simulink model "BDC_prototype"  (R2019a)
settings: Solver=VariableStepAuto  StartTime=0.0  StopTime=10.0  RelTol=1e-3
values from neighbouring files (symbols this model uses):
  sample_time = Ts    (= 0.0001)    [current_digital_control.m]    (also in voltage_digital_control.m)
undefined symbols (not defined in the file or in its folder): Ion, Lithium
libraries: powerlib x52, electricdrivelib x2, simulink x2, simulink_extras x1
settings Model: Creator=kagom  LastModifiedBy=kagom
settings SolverCC: ZeroCrossAlgorithm=Adaptive  AlgebraicLoopSolver=LineSearch
settings DebuggingCC: IgnoredZcDiagnostic=none

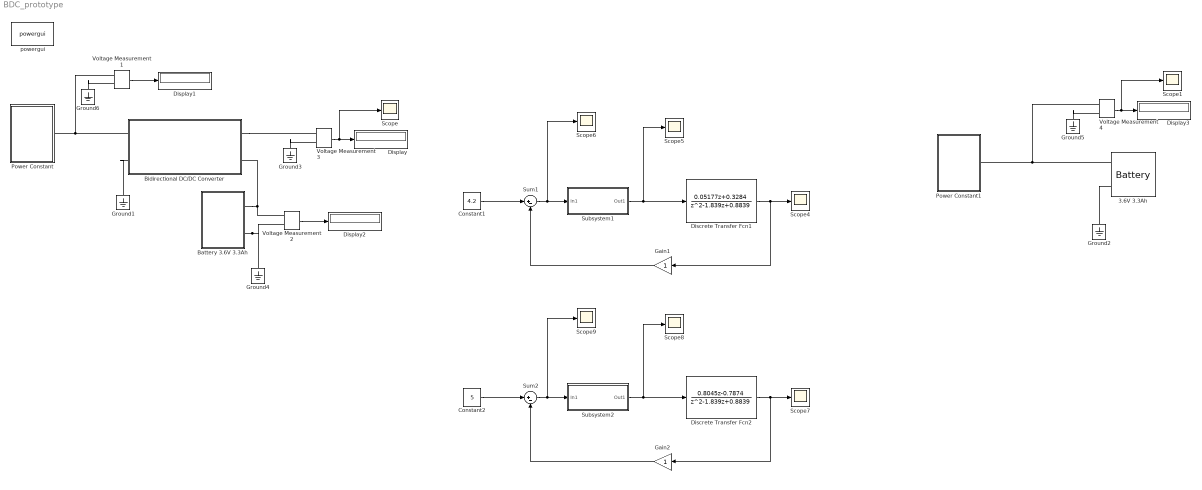
== system BDC_prototype ==
  3.6V 3.3Ah : electricdrivelib/Extra Sources/Battery  BatType=Lithium-Ion  ShowTempParam=off  ThermalPreset=no  ShowAgeParam=off  NomV=3.6  NomQ=3.3  SOC=20  Batt_Tr=1  PresetModel=on  MaxQ=3.3  MinV=2.7  FullV=4.1904  Dis_rate=1.4348  R=0.010909  Normal_OP=2.9843  expZone="[3.8894     0.16213]"  current=[6.5 13 32.5]  Units=Ampere-hour  Tci=20  NomT=20  T2=-30  MaxQ2=4.8  FullV2=7.1  Normal_OP2=5.655  expZone2="[6.58           1]"  Rca=0.6  ti=2000  Dp=0  Neq0=0  Tsim=1e6  Ta1=25  Qeol=5.4*0.9  Reol=0.013333*1.2  Char_age=[2.3478, 3]  Dis_age=[2.3478, 10]  N1=1500  N2=10500  N3=1000  N4=1400  Ta2=45  N5=950
      settings: SourceProductName=Simscape Electrical
  Battery 3.6V 3.3Ah : Subsystem
  Bidirectional DC/DC Converter : Subsystem
  Constant1 : Constant  Value=4.2  VectorParams1D=off
  Constant2 : Constant  Value=5  VectorParams1D=off
  Discrete Transfer Fcn1 : DiscreteTransferFcn  Numerator=[0.05177 0.3284]  Denominator=[1 -1.839 0.8839]
  Discrete Transfer Fcn2 : DiscreteTransferFcn  Numerator=[0.8045 -0.7874]  Denominator=[1 -1.839 0.8839]
  Display{,1..3} (4 alike) : Display
  Gain1 : Gain
  Gain2 : Gain
  Ground{1..6} (6 alike) : powerlib/Elements/Ground  LConnTagsString=a
      settings: SourceProductName=Simscape Electrical
  Power Constant : Subsystem
  Power Constant1 : Subsystem
  Scope{,1,4..9} (8 alike) : Scope
  Subsystem1 : Subsystem
  Subsystem2 : Subsystem
  Sum1 : Sum  Inputs=|+-
  Sum2 : Sum  Inputs=|+-
  Voltage Measurement{1..4} (4 alike) : powerlib/Measurements/Voltage Measurement  PhasorSimulation=off  OutputType=Complex  PSBequivalent=0
      settings: SourceProductName=Simscape Electrical
  powergui : powerlib/powergui  Priority=1  SimulationMode=Discrete  SampleTime=8e-6  frequency=60  Iterations=50  frequencyindice=0  Pbase=100e6  ErrMax=1e-4  UnitsV=kV  UnitsW=MW  buscounter=0  FunctionMessages=off  echomessages=off  EnableUseOfTLC=off  CurrentSourceSwitches=off  DisableSnubberDevices=off  DisableRonSwitches=off  DisableVfSwitches=off  DisplayEquations=off  AutomaticDiscreteSolvers=off  SolverType=Tustin/Backward Euler (TBE)  Interpol=off  ExternalGateDelay=off  methode=off  Ts=100  x0status=blocks  SPID=on  SwTol=0  HookPort=off  NonlinearTolerance=0  nMaxIteration=15  ContinueOnMaxIteration=off  RestoreLinks=warning  ResistiveCurrentMeasurement=off  Frange=[0:2:500]  Ylog=off  Xlog=on  ShowGrid=off  save=off  variable=ZData  structure=0  ZoomFFT=off  StartTime=0.0  cycles=1  DisplayStyle=1  fundamental=60  FreqAxis=off  MaxFrequency=1000  frequencyindicesteady=1  RmsSteady=1  display=off
      settings: SourceProductName=Simscape Electrical
  wires:
  Voltage Measurement1/1 -> Display1/1
  Voltage Measurement2/1 -> Display2/1
  Voltage Measurement3/1 -> Scope/1, Display/1
  Discrete Transfer Fcn1/1 -> Scope4/1, Gain1/1
  Gain1/1 -> Sum1/2
  Subsystem1/1(Out1) -> Scope5/1, Discrete Transfer Fcn1/1
  Sum1/1 -> Scope6/1, Subsystem1/1(In1)
  Constant1/1 -> Sum1/1
  Discrete Transfer Fcn2/1 -> Scope7/1, Gain2/1
  Subsystem2/1(Out1) -> Scope8/1, Discrete Transfer Fcn2/1
  Sum2/1 -> Scope9/1, Subsystem2/1(In1)
  Gain2/1 -> Sum2/2
  Constant2/1 -> Sum2/1
  Voltage Measurement4/1 -> Scope1/1, Display3/1
  connections:
  Voltage Measurement2/LConn1 -- Battery 3.6V 3.3Ah/RConn1 -- Bidirectional DC/DC Converter/RConn2
  Voltage Measurement1/LConn1 -- Bidirectional DC/DC Converter/LConn1 -- Power Constant/RConn1
  Battery 3.6V 3.3Ah/RConn2 -- Ground4/LConn1 -- Voltage Measurement2/LConn2
  Bidirectional DC/DC Converter/RConn1 -- Voltage Measurement3/LConn1
  Bidirectional DC/DC Converter/LConn2 -- Ground1/LConn1
  Ground6/LConn1 -- Voltage Measurement1/LConn2
  Ground3/LConn1 -- Voltage Measurement3/LConn2
  3.6V 3.3Ah/LConn1 -- Voltage Measurement4/LConn1 -- Power Constant1/RConn1
  Ground2/LConn1 -- 3.6V 3.3Ah/LConn2
  Ground5/LConn1 -- Voltage Measurement4/LConn2

== system BDC_prototype/Battery 3.6V 3.3Ah ==
  3.6V 3.3Ah : electricdrivelib/Extra Sources/Battery  BatType=Lithium-Ion  ShowTempParam=off  ThermalPreset=no  ShowAgeParam=off  NomV=3.6  NomQ=3.3  SOC=20  Batt_Tr=1  PresetModel=on  MaxQ=3.3  MinV=2.7  FullV=4.1904  Dis_rate=1.4348  R=0.010909  Normal_OP=2.9843  expZone="[3.8894     0.16213]"  current=[6.5 13 32.5]  Units=Ampere-hour  Tci=20  NomT=20  T2=-30  MaxQ2=4.8  FullV2=7.1  Normal_OP2=5.655  expZone2="[6.58           1]"  Rca=0.6  ti=2000  Dp=0  Neq0=0  Tsim=1e6  Ta1=25  Qeol=5.4*0.9  Reol=0.013333*1.2  Char_age=[2.3478, 3]  Dis_age=[2.3478, 10]  N1=1500  N2=10500  N3=1000  N4=1400  Ta2=45  N5=950
      settings: SourceProductName=Simscape Electrical
  Demux : Demux  Outputs=3
  + : PMIOPort  Side=Right
  GND : PMIOPort  Port=2  Side=Right
  tag scope: A=global, SOC=global, V=global
  wires:
  Demux/3 -> [V]
  3.6V 3.3Ah/1 -> Demux/1
  Demux/1 -> [SOC]
  Demux/2 -> [A]
  connections:
  3.6V 3.3Ah/LConn1 -- +/RConn1
  3.6V 3.3Ah/LConn2 -- GND/RConn1

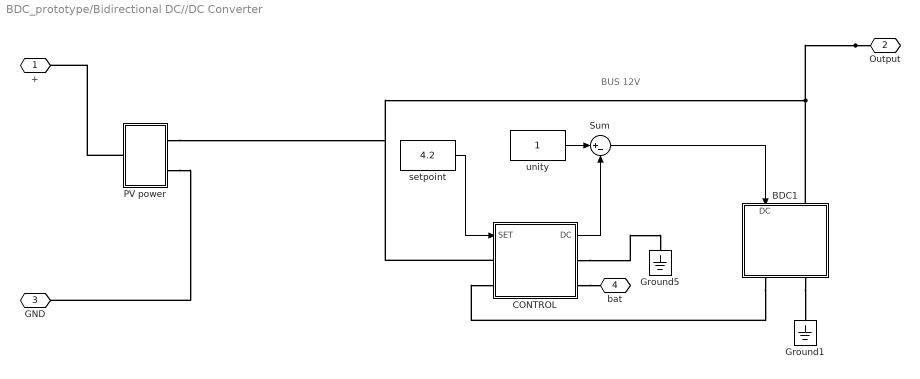
== system BDC_prototype/Bidirectional DC//DC Converter ==
  note: BUS 12V
  BDC1 : Subsystem  mask(BDC model){Ron=0.04, VD=1.5, RD=0.05, freq=125e3, tdead=19.125e-9, InputVariableName=bdc_in, OutputVariableName=bdc_out, SampleTime=sample_time}
      mask prompts: Ron "Mosfet On Resistance (Ohms)"; VD "Diode forward voltage (V)"; RD "Diode on resistance (Ohms)"; freq "Converter switching frequency (Hz)"; tdead "Driver dead time (s)"; InputVariableName "Input measurements variable name"; OutputVariableName "Output measurements variable name"; SampleTime "Simulink:blkprm_prompts:AllBlksSampleTime"
      mask help: Half-bridge averaged model with averaged losses.
      mask TypeOptions Ron: Driving Mosfet Loss/Ron | Sincronous Mosfet Loss/Ron
      mask TypeOptions VD: Diode Foward Voltage/VD
      mask TypeOptions RD: Diode On Resistance/RD
      mask TypeOptions freq:
      | Timing/fs/Value | Reverse Recovery
      | Loss of Lower Diode/freq | Reverse Recovery
      | Loss of Upper Diode/freq
      mask TypeOptions tdead: Timing/tdead/Value
      mask TypeOptions InputVariableName: Input_power/To Workspace/VariableName
      mask TypeOptions OutputVariableName: Output_power/To Workspace/VariableName
      mask TypeOptions SampleTime: Input_power/To Workspace/SampleTime | Output_power/To Workspace/SampleTime
      mask DialogControl Container9 Prompt: Logging
      mask DialogControl SampleTime Prompt: Sample time (-1 for inherited):
  CONTROL : Subsystem
  Ground1 : powerlib/Elements/Ground  LConnTagsString=a
      settings: SourceProductName=Simscape Electrical
  Ground5 : powerlib/Elements/Ground  LConnTagsString=a
      settings: SourceProductName=Simscape Electrical
  PV power : Subsystem
  Sum : Sum  Inputs=|+-
  setpoint : Constant  Value=4.2
  unity : Constant
  + : PMIOPort  Side=Left
  Output : PMIOPort  Port=2  Side=Right
  GND : PMIOPort  Port=3  Side=Left
  bat : PMIOPort  Port=4  Side=Right
  wires:
  setpoint/1 -> CONTROL/1(SET)
  Sum/1 -> BDC1/1(DC)
  CONTROL/1(DC) -> Sum/2
  unity/1 -> Sum/1
  connections:
  Output/RConn1 -- BDC1/LConn1 -- PV power/RConn1 -- CONTROL/LConn1
  CONTROL/RConn1 -- Ground5/LConn1
  BDC1/RConn2 -- Ground1/LConn1
  PV power/LConn1 -- +/RConn1
  PV power/RConn2 -- GND/RConn1
  BDC1/RConn1 -- CONTROL/LConn2
  CONTROL/RConn2 -- bat/RConn1

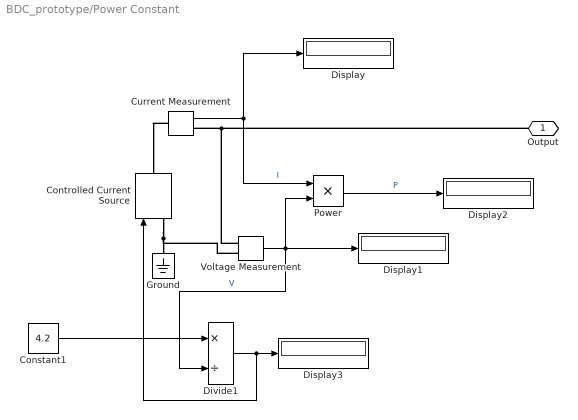
== system BDC_prototype/Power Constant ==
  Constant1 : Constant  Value=4.2  VectorParams1D=off
  Controlled Current Source : powerlib/Electrical Sources/Controlled Current Source  Initialize=on  Source_Type=DC  Amplitude=1  Phase=0  Frequency=0  Measurements=Current
      settings: SourceProductName=Simscape Electrical
  Current Measurement : powerlib/Measurements/Current Measurement  PhasorSimulation=off  OutputType=Complex  PSBequivalent=0
      settings: SourceProductName=Simscape Electrical
  Display{,1..3} (4 alike) : Display
  Divide1 : Product  Inputs=*/
  Ground : powerlib/Elements/Ground  LConnTagsString=a
      settings: SourceProductName=Simscape Electrical
  Power : Product
  Voltage Measurement : powerlib/Measurements/Voltage Measurement  PhasorSimulation=off  OutputType=Complex  PSBequivalent=0
      settings: SourceProductName=Simscape Electrical
  Output : PMIOPort  Side=Right
  wires:
  Voltage Measurement/1 -> Power/2, Divide1/2, Display1/1  "V"
  Current Measurement/1 -> Display/1, Power/1  "I"
  Power/1 -> Display2/1  "P"
  Divide1/1 -> Controlled Current Source/1, Display3/1
  Constant1/1 -> Divide1/1
  connections:
  Controlled Current Source/LConn1 -- Voltage Measurement/LConn2 -- Ground/LConn1
  Voltage Measurement/LConn1 -- Output/RConn1 -- Current Measurement/RConn1
  Current Measurement/LConn1 -- Controlled Current Source/RConn1

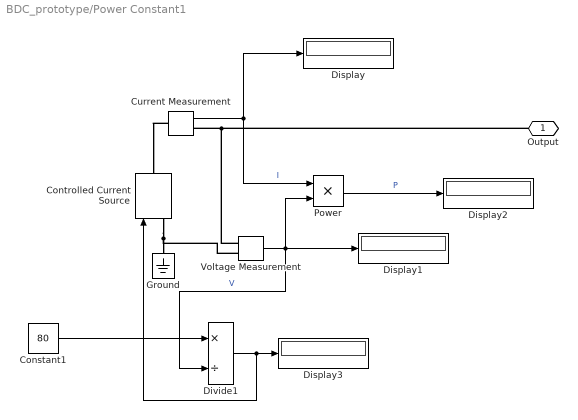
== system BDC_prototype/Power Constant1 ==
  Constant1 : Constant  Value=80  VectorParams1D=off
  Controlled Current Source : powerlib/Electrical Sources/Controlled Current Source  Initialize=on  Source_Type=DC  Amplitude=1  Phase=0  Frequency=0  Measurements=Current
      settings: SourceProductName=Simscape Electrical
  Current Measurement : powerlib/Measurements/Current Measurement  PhasorSimulation=off  OutputType=Complex  PSBequivalent=0
      settings: SourceProductName=Simscape Electrical
  Display{,1..3} (4 alike) : Display
  Divide1 : Product  Inputs=*/
  Ground : powerlib/Elements/Ground  LConnTagsString=a
      settings: SourceProductName=Simscape Electrical
  Power : Product
  Voltage Measurement : powerlib/Measurements/Voltage Measurement  PhasorSimulation=off  OutputType=Complex  PSBequivalent=0
      settings: SourceProductName=Simscape Electrical
  Output : PMIOPort  Side=Right
  wires:
  Voltage Measurement/1 -> Power/2, Divide1/2, Display1/1  "V"
  Current Measurement/1 -> Display/1, Power/1  "I"
  Power/1 -> Display2/1  "P"
  Divide1/1 -> Controlled Current Source/1, Display3/1
  Constant1/1 -> Divide1/1
  connections:
  Controlled Current Source/LConn1 -- Voltage Measurement/LConn2 -- Ground/LConn1
  Voltage Measurement/LConn1 -- Output/RConn1 -- Current Measurement/RConn1
  Current Measurement/LConn1 -- Controlled Current Source/RConn1

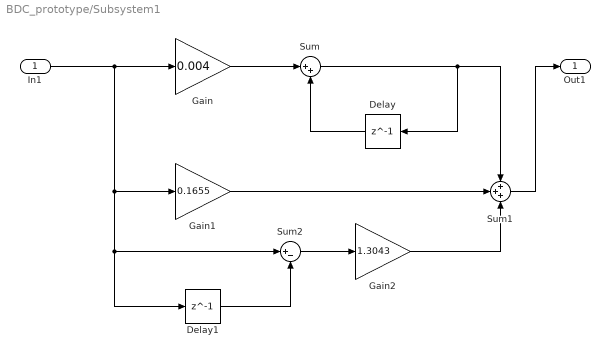
== system BDC_prototype/Subsystem1 ==
  In1 : Inport
  Delay : Delay  DelayLength=1
  Delay1 : Delay  DelayLength=1
  Gain : Gain  Gain=0.004
  Gain1 : Gain  Gain=0.1655
  Gain2 : Gain  Gain=1.3043
  Sum : Sum  Inputs=|++
  Sum1 : Sum  Inputs=+++
  Sum2 : Sum  Inputs=|+-
  Out1 : Outport
  wires:
  Gain/1 -> Sum/1
  Delay/1 -> Sum/2
  Sum/1 -> Delay/1, Sum1/1
  In1/1 -> Sum2/1, Delay1/1, Gain1/1, Gain/1
  Gain1/1 -> Sum1/2
  Delay1/1 -> Sum2/2
  Sum2/1 -> Gain2/1
  Gain2/1 -> Sum1/3
  Sum1/1 -> Out1/1

== system BDC_prototype/Subsystem2 ==
  In1 : Inport
  Delay : Delay  DelayLength=1
  Gain : Gain  Gain=0.2452
  Gain1 : Gain  Gain=0.6566
  Sum : Sum  Inputs=|++
  Sum1 : Sum
  Out1 : Outport
  wires:
  Gain/1 -> Sum/1
  Delay/1 -> Sum/2
  Sum/1 -> Delay/1, Sum1/1
  In1/1 -> Gain1/1, Gain/1
  Sum1/1 -> Out1/1
  Gain1/1 -> Sum1/2

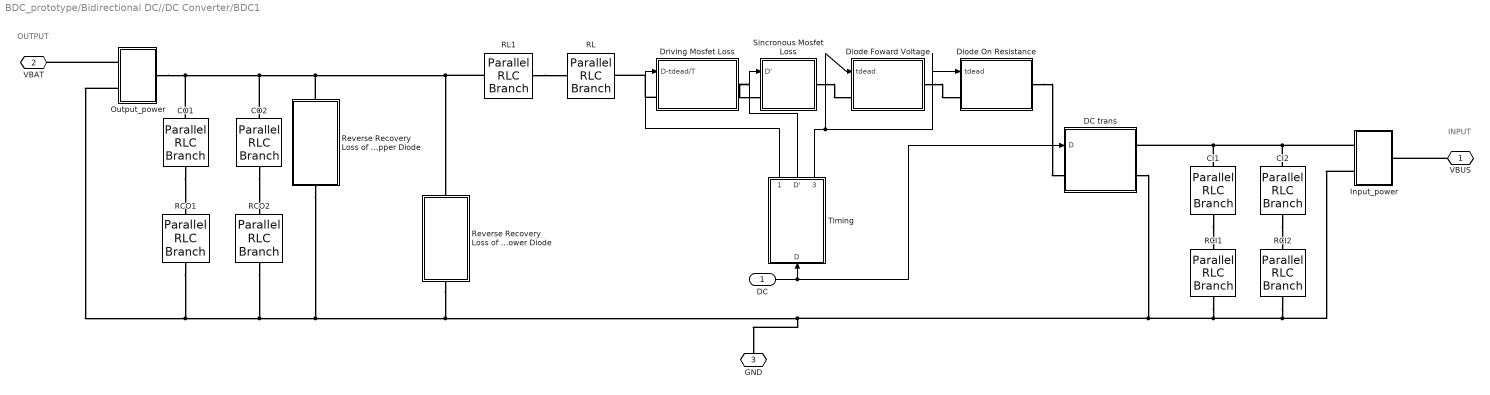
== system BDC_prototype/Bidirectional DC//DC Converter/BDC1 ==
  note: INPUT
  note: OUTPUT
  DC : Inport
  CI1 : powerlib/Elements/Parallel RLC Branch  LConnTagsString=a  RConnTagsString=__new0  BranchType=C  Resistance=7  Inductance=1e-3  SetiL0=off  InitialCurrent=0  Capacitance=33e-6  Setx0=off  InitialVoltage=10  Measurements=None
      settings: SourceProductName=Simscape Electrical
  CI2 : powerlib/Elements/Parallel RLC Branch  LConnTagsString=a  RConnTagsString=__new0  BranchType=C  Resistance=7  Inductance=1e-3  SetiL0=off  InitialCurrent=0  Capacitance=1e-6  Setx0=off  InitialVoltage=10  Measurements=None
      settings: SourceProductName=Simscape Electrical
  CO1 : powerlib/Elements/Parallel RLC Branch  LConnTagsString=a  RConnTagsString=__new0  BranchType=C  Resistance=7  Inductance=1e-3  SetiL0=off  InitialCurrent=0  Capacitance=33e-6  Setx0=off  InitialVoltage=10  Measurements=None
      settings: SourceProductName=Simscape Electrical
  CO2 : powerlib/Elements/Parallel RLC Branch  LConnTagsString=a  RConnTagsString=__new0  BranchType=C  Resistance=7  Inductance=1e-3  SetiL0=off  InitialCurrent=0  Capacitance=1e-6  Setx0=off  InitialVoltage=10  Measurements=None
      settings: SourceProductName=Simscape Electrical
  DC trans : Subsystem
      mask Display: text(0.5,0.5,'1 : {\itD}','horizontalAlignment', 'center', 'verticalAlignment','middle','texmode','on')
  Diode Foward Voltage : Subsystem  mask{VD=VD}
      mask prompts: VD "Diode forward voltage (V)"
      mask Display: text(0.5,0.5,'{\itt_{dead}\cdotT^{ -1}}\cdot{\itV_{D}}','horizontalAlignment', 'center', 'verticalAlignment','middle','texmode','on')
  Diode On Resistance : Subsystem  mask{RD=RD}
      mask prompts: RD "Diode on resistance (Ohms)"
      mask Display: text(0.5,0.5,'{\itt_{dead}\cdotT^{ -1}}\cdot{\itR_{D}}','horizontalAlignment', 'center', 'verticalAlignment','middle','texmode','on')
  Driving Mosfet Loss : Subsystem  mask{Ron=Ron}
      mask prompts: Ron "Mosfet On Resistance (Ohms)"
      mask Display: text(0.5,0.5,'({\itD - t_{dead}\cdotT^{ -1}})\cdot{\itR_{on}}','horizontalAlignment', 'center', 'verticalAlignment','middle','texmode','on')
  Input_power : Subsystem
  Output_power : Subsystem
  RCI1 : powerlib/Elements/Parallel RLC Branch  LConnTagsString=a  RConnTagsString=__new0  BranchType=R  Resistance=40e-3  Inductance=1e-3  SetiL0=off  InitialCurrent=0  Capacitance=100e-6  Setx0=off  InitialVoltage=10  Measurements=None
      settings: SourceProductName=Simscape Electrical
  RCI2 : powerlib/Elements/Parallel RLC Branch  LConnTagsString=a  RConnTagsString=__new0  BranchType=R  Resistance=40e-3  Inductance=1e-3  SetiL0=off  InitialCurrent=0  Capacitance=100e-6  Setx0=off  InitialVoltage=10  Measurements=None
      settings: SourceProductName=Simscape Electrical
  RCO1 : powerlib/Elements/Parallel RLC Branch  LConnTagsString=a  RConnTagsString=__new0  BranchType=R  Resistance=40e-3  Inductance=1e-3  SetiL0=off  InitialCurrent=0  Capacitance=100e-6  Setx0=off  InitialVoltage=10  Measurements=None
      settings: SourceProductName=Simscape Electrical
  RCO2 : powerlib/Elements/Parallel RLC Branch  LConnTagsString=a  RConnTagsString=__new0  BranchType=R  Resistance=40e-3  Inductance=1e-3  SetiL0=off  InitialCurrent=0  Capacitance=100e-6  Setx0=off  InitialVoltage=10  Measurements=None
      settings: SourceProductName=Simscape Electrical
  RL : powerlib/Elements/Parallel RLC Branch  LConnTagsString=a  RConnTagsString=__new0  BranchType=R  Resistance=43e-3  Inductance=50e-6  SetiL0=off  InitialCurrent=0  Capacitance=10e6/3  Setx0=off  InitialVoltage=0  Measurements=None
      settings: SourceProductName=Simscape Electrical
  RL1 : powerlib/Elements/Parallel RLC Branch  LConnTagsString=a  RConnTagsString=__new0  BranchType=L  Resistance=43e-3  Inductance=22e-6  SetiL0=off  InitialCurrent=0  Capacitance=10e6/3  Setx0=off  InitialVoltage=0  Measurements=None
      settings: SourceProductName=Simscape Electrical
  Reverse Recovery Loss of Lower Diode : Subsystem  mask{Qrr=65e-9, freq=freq}
      mask prompts: Qrr "Reverse recovery charge (C)"; freq "Converter switching frequency (Hz)"
      mask Display: text(0.5,0.5,'{\itQ_{rr}}\cdot{\itf_{sw}}','horizontalAlignment', 'center', 'verticalAlignment','middle','texmode','on')
  Reverse Recovery Loss of Upper Diode : Subsystem  mask{Qrr=65e-9, freq=freq}
      mask prompts: Qrr "Reverse recovery charge (C)"; freq "Converter switching frequency (Hz)"
      mask Display: text(0.5,0.5,'{\itQ_{rr}}\cdot{\itf_{sw}}','horizontalAlignment', 'center', 'verticalAlignment','middle','texmode','on')
  Sincronous Mosfet Loss : Subsystem  mask{Ron=Ron}
      mask prompts: Ron "Mosfet On Resistance (Ohms)"
      mask Display: text(0.5,0.5,'{\itD\prime}\cdot{\itR_{on}}','horizontalAlignment', 'center', 'verticalAlignment','middle','texmode','on')
  Timing : Subsystem
  "VBUS " : PMIOPort  Side=Left
  VBAT : PMIOPort  Port=2  Side=Right
  GND : PMIOPort  Port=3  Side=Right
  wires:
  DC/1 -> DC trans/1(D), Timing/1(D)
  Timing/3(tdead/T) -> Diode On Resistance/1(tdead), Diode Foward Voltage/1(tdead)
  Timing/1(D - tdead/Ts) -> Driving Mosfet Loss/1(D-tdead/T)
  Timing/2(D') -> Sincronous Mosfet Loss/1(D')
  connections:
  DC trans/RConn2 -- RCI2/RConn1 -- Input_power/RConn2 -- RCI1/RConn1 -- RCO2/RConn1 -- RCO1/RConn1 -- Output_power/RConn2 -- Reverse Recovery Loss of Upper Diode/LConn1 -- Reverse Recovery Loss of Lower Diode/LConn1 -- GND/RConn1
  Driving Mosfet Loss/LConn1 -- RL/RConn1
  Driving Mosfet Loss/RConn1 -- Sincronous Mosfet Loss/LConn1
  Sincronous Mosfet Loss/RConn1 -- Diode Foward Voltage/LConn1
  Diode Foward Voltage/RConn1 -- Diode On Resistance/LConn1
  Diode On Resistance/RConn1 -- DC trans/LConn1
  CO1/LConn1 -- CO2/LConn1 -- RL1/LConn1 -- Reverse Recovery Loss of Lower Diode/RConn1 -- Reverse Recovery Loss of Upper Diode/RConn1 -- Output_power/LConn1
  CI1/LConn1 -- CI2/LConn1 -- Input_power/RConn1 -- DC trans/RConn1
  CI1/RConn1 -- RCI1/LConn1
  CO1/RConn1 -- RCO1/LConn1
  "VBUS "/RConn1 -- Input_power/LConn1
  Output_power/RConn1 -- VBAT/RConn1
  CO2/RConn1 -- RCO2/LConn1
  CI2/RConn1 -- RCI2/LConn1
  RL1/RConn1 -- RL/LConn1

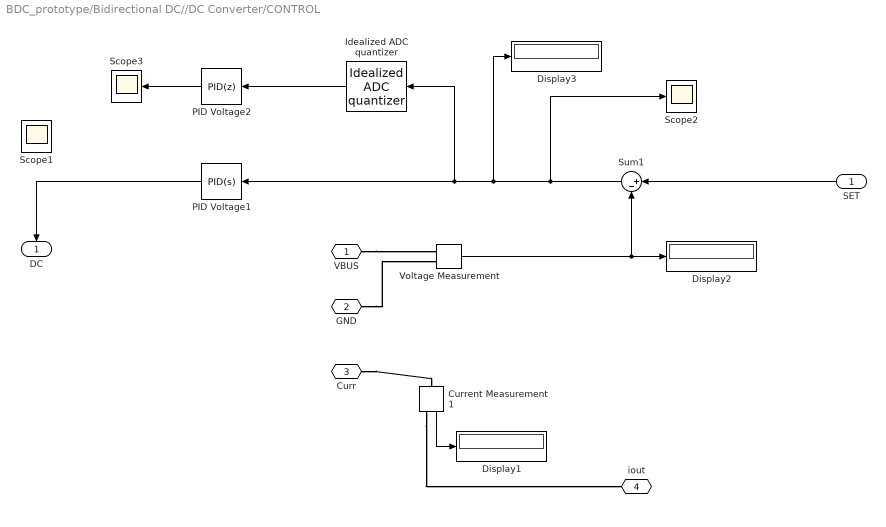
== system BDC_prototype/Bidirectional DC//DC Converter/CONTROL ==
  SET : Inport
  Current Measurement1 : powerlib/Measurements/Current Measurement  PhasorSimulation=off  OutputType=Complex  PSBequivalent=0
      settings: SourceProductName=Simscape Electrical
  Display1 : Display
  Display2 : Display
  Display3 : Display
  Idealized ADC quantizer : simulink_extras/Additional Discrete/Idealized ADC quantizer  NumberOfConverterBits=12  Vmin=0  Vmax=5  OutputDataType=double  OutputNegativeValues=off
      settings: SourceProductName=Simulink
  PID Voltage1 : simulink/Continuous/PID Controller  Controller=PID  Form=Parallel  TimeDomain=Continuous-time  SampleTime=-1  IntegratorMethod=Backward Euler  FilterMethod=Forward Euler  ControllerParametersSource=internal  P=0.1113  I=0.0022  D=1.3378  UseFilter=on  N=1000  TunerSelectOption=Transfer Function Based (PID Tuner App)  InitialConditionSource=internal  InitialConditionForIntegrator=0  InitialConditionForFilter=0  DifferentiatorICPrevScaledInput=0  ExternalReset=none  TrackingMode=off  Kt=1  LimitOutput=on  UpperSaturationLimit=0.95  LowerSaturationLimit=0.05  LinearizeAsGain=off  AntiWindupMode=none  Kb=1  POutMin=[]  POutMax=[]  IOutMin=[]  IOutMax=[]  DOutMin=[]  DOutMax=[]  NOutMin=[]  NOutMax=[]  SumOutMin=[]  SumOutMax=[]  SaturationOutMin=[]  SaturationOutMax=[]  PParamMin=[]  PParamMax=[]  IParamMin=[]  IParamMax=[]  DParamMin=[]  DParamMax=[]  NParamMin=[]  NParamMax=[]  KbParamMin=[]  KbParamMax=[]  KtParamMin=[]  KtParamMax=[]  KbOutMin=[]  KbOutMax=[]  KtOutMin=[]  KtOutMax=[]  IntegratorOutMin=[]  IntegratorOutMax=[]  FilterOutMin=[]  FilterOutMax=[]  SumI1OutMin=[]  SumI1OutMax=[]  SumI2OutMin=[]  SumI2OutMax=[]  SumI3OutMin=[]  SumI3OutMax=[]  SumI4OutMin=[]  SumI4OutMax=[]  SumDOutMin=[]  SumDOutMax=[]  DifferentiatorOutMin=[]  DifferentiatorOutMax=[]  FilterDiffOutCoefMin=[]  FilterDiffOutCoefMax=[]  ReciprocalOutMin=[]  ReciprocalOutMax=[]  SumDenOutMin=[]  SumDenOutMax=[]  SumNumOutMin=[]  SumNumOutMax=[]  DivideOutMin=[]  DivideOutMax=[]  IntegratorContinuousStateAttributes=''  IntegratorStateMustResolveToSignalObject=off  IntegratorRTWStateStorageClass=Auto  FilterContinuousStateAttributes=''  FilterStateMustResolveToSignalObject=off  FilterRTWStateStorageClass=Auto  ParallelPVariant=InternalParameters  IdealPVariant=Disabled  IVariant=InternalParameters  DVariant=InternalParameters  IntegratorVariant=Continuous  SatVariant=Enabled  AWVariant=Passthrough  PCopyVariant=Disabled  TRVariant=Disabled  FdbkBlocksVariant=Forward  IdealPFdbkVariant=Disabled  SatFdbkVariant=Disabled  DerivativeFilterVariant=ContFilter  NVariant=InternalParameters  NCopyVariant=Disabled  FilterICVariant=InternalICsFilter  IntegratorICVariant=InternalICs  ExternalResetVariant=Disabled  TRSumVariant=Passthrough  SumFdbkVariant=Disabled  SumVariant=Sum_PID
  PID Voltage2 : simulink/Continuous/PID Controller  Controller=PID  Form=Parallel  TimeDomain=Discrete-time  SampleTime=-1  IntegratorMethod=Backward Euler  FilterMethod=Forward Euler  ControllerParametersSource=internal  P=0.0440  I=0.000193  D=1.1886  UseFilter=on  N=1000  TunerSelectOption=Transfer Function Based (PID Tuner App)  InitialConditionSource=internal  InitialConditionForIntegrator=0  InitialConditionForFilter=0  DifferentiatorICPrevScaledInput=0  ExternalReset=none  TrackingMode=off  Kt=1  LimitOutput=on  UpperSaturationLimit=0.95  LowerSaturationLimit=0.05  LinearizeAsGain=off  AntiWindupMode=none  Kb=1  POutMin=[]  POutMax=[]  IOutMin=[]  IOutMax=[]  DOutMin=[]  DOutMax=[]  NOutMin=[]  NOutMax=[]  SumOutMin=[]  SumOutMax=[]  SaturationOutMin=[]  SaturationOutMax=[]  PParamMin=[]  PParamMax=[]  IParamMin=[]  IParamMax=[]  DParamMin=[]  DParamMax=[]  NParamMin=[]  NParamMax=[]  KbParamMin=[]  KbParamMax=[]  KtParamMin=[]  KtParamMax=[]  KbOutMin=[]  KbOutMax=[]  KtOutMin=[]  KtOutMax=[]  IntegratorOutMin=[]  IntegratorOutMax=[]  FilterOutMin=[]  FilterOutMax=[]  SumI1OutMin=[]  SumI1OutMax=[]  SumI2OutMin=[]  SumI2OutMax=[]  SumI3OutMin=[]  SumI3OutMax=[]  SumI4OutMin=[]  SumI4OutMax=[]  SumDOutMin=[]  SumDOutMax=[]  DifferentiatorOutMin=[]  DifferentiatorOutMax=[]  FilterDiffOutCoefMin=[]  FilterDiffOutCoefMax=[]  ReciprocalOutMin=[]  ReciprocalOutMax=[]  SumDenOutMin=[]  SumDenOutMax=[]  SumNumOutMin=[]  SumNumOutMax=[]  DivideOutMin=[]  DivideOutMax=[]  IntegratorContinuousStateAttributes=''  IntegratorStateMustResolveToSignalObject=off  IntegratorRTWStateStorageClass=Auto  FilterContinuousStateAttributes=''  FilterStateMustResolveToSignalObject=off  FilterRTWStateStorageClass=Auto  ParallelPVariant=InternalParameters  IdealPVariant=Disabled  IVariant=InternalParameters  DVariant=InternalParameters  IntegratorVariant=Discrete  SatVariant=Enabled  AWVariant=Passthrough  PCopyVariant=Disabled  TRVariant=Disabled  FdbkBlocksVariant=Forward  IdealPFdbkVariant=Disabled  SatFdbkVariant=Disabled  DerivativeFilterVariant=ForwardEulerFilter  NVariant=InternalParameters  NCopyVariant=Disabled  FilterICVariant=InternalICsFilter  IntegratorICVariant=InternalICs  ExternalResetVariant=Disabled  TRSumVariant=Passthrough  SumFdbkVariant=Disabled  SumVariant=Sum_PID
  Scope1 : Scope
  Scope2 : Scope
  Scope3 : Scope
  Sum1 : Sum  Inputs=|+-
  Voltage Measurement : powerlib/Measurements/Voltage Measurement  PhasorSimulation=off  OutputType=Complex  PSBequivalent=0
      settings: SourceProductName=Simscape Electrical
  VBUS : PMIOPort  Side=Left
  GND : PMIOPort  Port=2  Side=Right
  Curr : PMIOPort  Port=3  Side=Left
  iout : PMIOPort  Port=4  Side=Right
  DC : Outport
  wires:
  Voltage Measurement/1 -> Display2/1, Sum1/2
  Current Measurement1/1 -> Display1/1
  SET/1 -> Sum1/1
  Sum1/1 -> Display3/1, Idealized ADC quantizer/1, PID Voltage1/1, Scope2/1
  Idealized ADC quantizer/1 -> PID Voltage2/1
  PID Voltage2/1 -> Scope3/1
  PID Voltage1/1 -> DC/1
  connections:
  VBUS/RConn1 -- Voltage Measurement/LConn1
  GND/RConn1 -- Voltage Measurement/LConn2
  Current Measurement1/RConn1 -- iout/RConn1
  Curr/RConn1 -- Current Measurement1/LConn1

== system BDC_prototype/Bidirectional DC//DC Converter/PV power ==
  Bus Creator : BusCreator  Inputs=3
  Current Measurement : powerlib/Measurements/Current Measurement  PhasorSimulation=off  OutputType=Complex  PSBequivalent=0
      settings: SourceProductName=Simscape Electrical
  Power : Product
  Voltage Measurement : powerlib/Measurements/Voltage Measurement  PhasorSimulation=off  OutputType=Complex  PSBequivalent=0
      settings: SourceProductName=Simscape Electrical
  + : PMIOPort  Side=Left
  - : PMIOPort  Port=2  Side=Right
  REF : PMIOPort  Port=3  Side=Right
  wires:
  Bus Creator/1 -> ?
  Voltage Measurement/1 -> Bus Creator/2, Power/2  "V"
  Current Measurement/1 -> Bus Creator/1, Power/1  "I"
  Power/1 -> Bus Creator/3  "P"
  connections:
  Voltage Measurement/LConn2 -- REF/RConn1
  Current Measurement/RConn1 -- -/RConn1
  Current Measurement/LConn1 -- Voltage Measurement/LConn1 -- +/RConn1

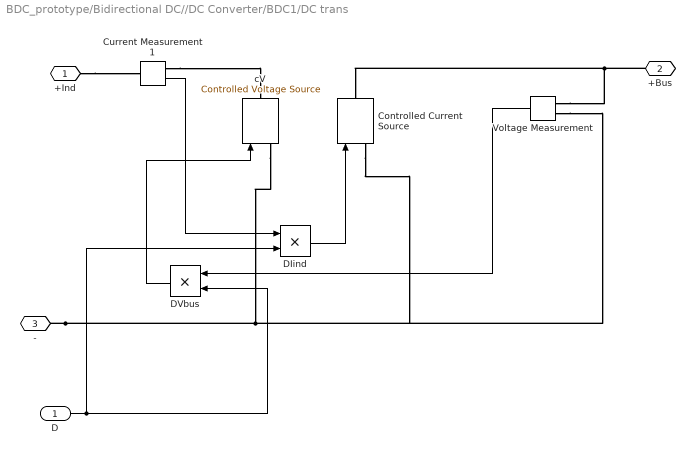
== system BDC_prototype/Bidirectional DC//DC Converter/BDC1/DC trans ==
  D : Inport
  Controlled Current Source : powerlib/Electrical Sources/Controlled Current Source  Initialize=on  Source_Type=DC  Amplitude=0  Phase=0  Frequency=0  Measurements=None
      settings: SourceProductName=Simscape Electrical
  Current Measurement1 : powerlib/Measurements/Current Measurement  PhasorSimulation=off  OutputType=Complex  PSBequivalent=0
      settings: SourceProductName=Simscape Electrical
  DIind : Product
  DVbus : Product
  Voltage Measurement : powerlib/Measurements/Voltage Measurement  PhasorSimulation=off  OutputType=Complex  PSBequivalent=0
      settings: SourceProductName=Simscape Electrical
  cV : powerlib/Electrical Sources/Controlled Voltage Source  Initialize=on  Source_Type=DC  Amplitude=0  Phase=0  Frequency=0  Measurements=None
      settings: SourceProductName=Simscape Electrical
  +Ind : PMIOPort  Side=Left
  +Bus : PMIOPort  Port=2  Side=Right
  - : PMIOPort  Port=3  Side=Right
  wires:
  D/1 -> DVbus/2, DIind/2
  Current Measurement1/1 -> DIind/1
  Voltage Measurement/1 -> DVbus/1
  DIind/1 -> Controlled Current Source/1
  DVbus/1 -> cV/1
  connections:
  Current Measurement1/RConn1 -- cV/RConn1
  -/RConn1 -- Controlled Current Source/LConn1 -- Voltage Measurement/LConn2 -- cV/LConn1
  +Ind/RConn1 -- Current Measurement1/LConn1
  +Bus/RConn1 -- Controlled Current Source/RConn1 -- Voltage Measurement/LConn1

== system BDC_prototype/Bidirectional DC//DC Converter/BDC1/Diode Foward Voltage ==
  tdead : Inport
  Constant : Constant  Value=VD
  Controlled Voltage Source : powerlib/Electrical Sources/Controlled Voltage Source  Initialize=on  Source_Type=AC  Amplitude=0  Phase=0  Frequency=0  Measurements=None
      settings: SourceProductName=Simscape Electrical
  Product1 : Product
  - : PMIOPort  Side=Right
  + : PMIOPort  Port=2  Side=Left
  wires:
  Constant/1 -> Product1/1
  Product1/1 -> Controlled Voltage Source/1
  tdead/1 -> Product1/2
  connections:
  Controlled Voltage Source/LConn1 -- -/RConn1
  +/RConn1 -- Controlled Voltage Source/RConn1

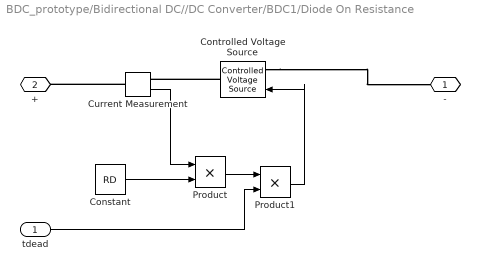
== system BDC_prototype/Bidirectional DC//DC Converter/BDC1/Diode On Resistance ==
  tdead : Inport
  Constant : Constant  Value=RD
  Controlled Voltage Source : powerlib/Electrical Sources/Controlled Voltage Source  Initialize=on  Source_Type=AC  Amplitude=0  Phase=0  Frequency=0  Measurements=None
      settings: SourceProductName=Simscape Electrical
  Current Measurement : powerlib/Measurements/Current Measurement  PhasorSimulation=off  OutputType=Complex  PSBequivalent=0
      settings: SourceProductName=Simscape Electrical
  Product : Product
  Product1 : Product
  - : PMIOPort  Side=Right
  + : PMIOPort  Port=2  Side=Left
  wires:
  Current Measurement/1 -> Product/1
  Constant/1 -> Product/2
  Product/1 -> Product1/1
  Product1/1 -> Controlled Voltage Source/1
  tdead/1 -> Product1/2
  connections:
  Current Measurement/LConn1 -- +/RConn1
  Controlled Voltage Source/LConn1 -- -/RConn1
  Controlled Voltage Source/RConn1 -- Current Measurement/RConn1

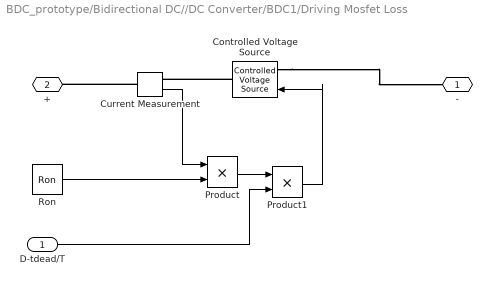
== system BDC_prototype/Bidirectional DC//DC Converter/BDC1/Driving Mosfet Loss ==
  D-tdead/T : Inport
  Controlled Voltage Source : powerlib/Electrical Sources/Controlled Voltage Source  Initialize=on  Source_Type=DC  Amplitude=0  Phase=0  Frequency=0  Measurements=None
      settings: SourceProductName=Simscape Electrical
  Current Measurement : powerlib/Measurements/Current Measurement  PhasorSimulation=off  OutputType=Complex  PSBequivalent=0
      settings: SourceProductName=Simscape Electrical
  Product : Product
  Product1 : Product
  Ron : Constant  Value=Ron
  - : PMIOPort  Side=Right
  + : PMIOPort  Port=2  Side=Left
  wires:
  D-tdead/T/1 -> Product1/2
  Current Measurement/1 -> Product/1
  Ron/1 -> Product/2
  Product/1 -> Product1/1
  Product1/1 -> Controlled Voltage Source/1
  connections:
  Current Measurement/LConn1 -- +/RConn1
  Controlled Voltage Source/LConn1 -- -/RConn1
  Controlled Voltage Source/RConn1 -- Current Measurement/RConn1

== system BDC_prototype/Bidirectional DC//DC Converter/BDC1/Input_power ==
  Bus Creator : BusCreator  Inputs=3
  Current Measurement : powerlib/Measurements/Current Measurement  PhasorSimulation=off  OutputType=Complex  PSBequivalent=0
      settings: SourceProductName=Simscape Electrical
  Power : Product
  Voltage Measurement : powerlib/Measurements/Voltage Measurement  PhasorSimulation=off  OutputType=Complex  PSBequivalent=0
      settings: SourceProductName=Simscape Electrical
  + : PMIOPort  Side=Left
  - : PMIOPort  Port=2  Side=Right
  REF : PMIOPort  Port=3  Side=Right
  wires:
  Voltage Measurement/1 -> Bus Creator/2, Power/2  "V"
  Current Measurement/1 -> Bus Creator/1, Power/1  "I"
  Power/1 -> Bus Creator/3  "P"
  connections:
  Voltage Measurement/LConn2 -- REF/RConn1
  Current Measurement/RConn1 -- -/RConn1
  Current Measurement/LConn1 -- Voltage Measurement/LConn1 -- +/RConn1

== system BDC_prototype/Bidirectional DC//DC Converter/BDC1/Output_power ==
  Bus Creator : BusCreator  Inputs=3
  Current Measurement : powerlib/Measurements/Current Measurement  PhasorSimulation=off  OutputType=Complex  PSBequivalent=0
      settings: SourceProductName=Simscape Electrical
  Power : Product
  Voltage Measurement : powerlib/Measurements/Voltage Measurement  PhasorSimulation=off  OutputType=Complex  PSBequivalent=0
      settings: SourceProductName=Simscape Electrical
  + : PMIOPort  Side=Left
  - : PMIOPort  Port=2  Side=Right
  REF : PMIOPort  Port=3  Side=Right
  wires:
  Voltage Measurement/1 -> Bus Creator/2, Power/2  "V"
  Current Measurement/1 -> Bus Creator/1, Power/1  "I"
  Power/1 -> Bus Creator/3  "P"
  connections:
  Voltage Measurement/LConn2 -- REF/RConn1
  Current Measurement/RConn1 -- -/RConn1
  Voltage Measurement/LConn1 -- +/RConn1 -- Current Measurement/LConn1

== system BDC_prototype/Bidirectional DC//DC Converter/BDC1/Reverse Recovery Loss of Lower Diode ==
  Constant : Constant  Value=0.5*Qrr*freq
  Reverse recovery : powerlib/Electrical Sources/Controlled Current Source  Initialize=on  Source_Type=AC  Amplitude=0  Phase=0  Frequency=0  Measurements=None
      settings: SourceProductName=Simscape Electrical
  + : PMIOPort  Side=Right
  - : PMIOPort  Port=2  Side=Left
  wires:
  Constant/1 -> Reverse recovery/1
  connections:
  Reverse recovery/LConn1 -- +/RConn1
  Reverse recovery/RConn1 -- -/RConn1

== system BDC_prototype/Bidirectional DC//DC Converter/BDC1/Reverse Recovery Loss of Upper Diode ==
  Constant : Constant  Value=0.5*Qrr*freq
  Reverse recovery : powerlib/Electrical Sources/Controlled Current Source  Initialize=on  Source_Type=AC  Amplitude=0  Phase=0  Frequency=0  Measurements=None
      settings: SourceProductName=Simscape Electrical
  + : PMIOPort  Side=Right
  - : PMIOPort  Port=2  Side=Left
  wires:
  Constant/1 -> Reverse recovery/1
  connections:
  Reverse recovery/RConn1 -- -/RConn1
  Reverse recovery/LConn1 -- +/RConn1

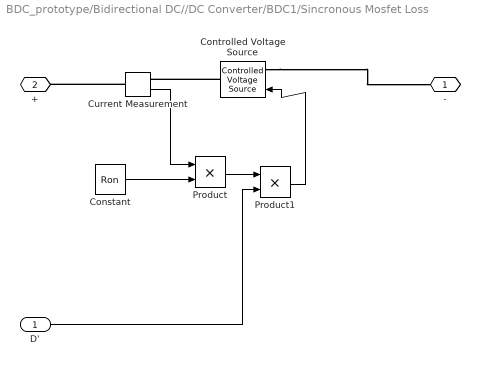
== system BDC_prototype/Bidirectional DC//DC Converter/BDC1/Sincronous Mosfet Loss ==
  D' : Inport
  Constant : Constant  Value=Ron
  Controlled Voltage Source : powerlib/Electrical Sources/Controlled Voltage Source  Initialize=on  Source_Type=DC  Amplitude=0  Phase=0  Frequency=0  Measurements=None
      settings: SourceProductName=Simscape Electrical
  Current Measurement : powerlib/Measurements/Current Measurement  PhasorSimulation=off  OutputType=Complex  PSBequivalent=0
      settings: SourceProductName=Simscape Electrical
  Product : Product
  Product1 : Product
  - : PMIOPort  Side=Right
  + : PMIOPort  Port=2  Side=Left
  wires:
  Product/1 -> Product1/1
  Constant/1 -> Product/2
  Current Measurement/1 -> Product/1
  Product1/1 -> Controlled Voltage Source/1
  D'/1 -> Product1/2
  connections:
  Controlled Voltage Source/RConn1 -- Current Measurement/RConn1
  Controlled Voltage Source/LConn1 -- -/RConn1
  Current Measurement/LConn1 -- +/RConn1

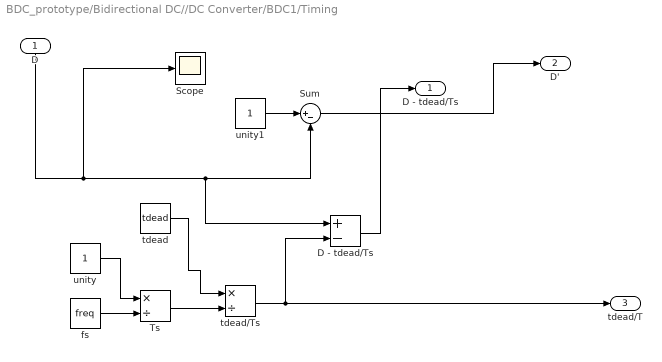
== system BDC_prototype/Bidirectional DC//DC Converter/BDC1/Timing ==
  D : Inport
  "D - tdead/Ts " : Sum  Inputs=+-
  Scope : Scope
  Sum : Sum  Inputs=|+-
  Ts : Product  Inputs=*/
  fs : Constant  Value=freq
  tdead : Constant  Value=tdead
  tdead/Ts : Product  Inputs=*/
  unity : Constant
  unity1 : Constant
  D - tdead/Ts : Outport
  D' : Outport  Port=2
  tdead/T : Outport  Port=3
  wires:
  unity/1 -> Ts/1
  tdead/1 -> tdead/Ts/1
  "D - tdead/Ts "/1 -> D - tdead/Ts/1
  fs/1 -> Ts/2
  Ts/1 -> tdead/Ts/2
  tdead/Ts/1 -> tdead/T/1, "D - tdead/Ts "/2
  unity1/1 -> Sum/1
  Sum/1 -> D'/1
  D/1 -> Scope/1, Sum/2, "D - tdead/Ts "/1
